simulink model "simulation_impulse"  (R2023b)
settings: Solver=VariableStepAuto  StartTime=0.0  StopTime=t_end  RelTol=1e-3
InitFcn:
  | param = plant_param();
undefined symbols (not defined in the file or in its folder): ue, xe
settings Model: Creator=block  LastModifiedBy=block

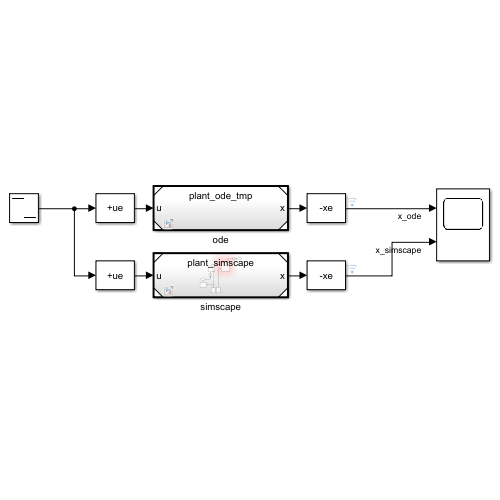
[thumbnail: Simulink's stored preview of the top-level diagram]
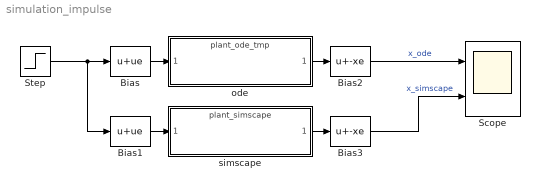
== system simulation_impulse ==
  Bias : Bias  Bias=ue  SaturateOnIntegerOverflow=off
  Bias1 : Bias  Bias=ue  SaturateOnIntegerOverflow=off
  Bias2 : Bias  Bias=-xe  SaturateOnIntegerOverflow=off
  Bias3 : Bias  Bias=-xe  SaturateOnIntegerOverflow=off
  Scope : Scope  NumInputPorts=2
  Step : Step  Time=0.01  Before=100  After=0  SampleTime=0
  ode : ModelReference  ModelNameDialog=plant_ode_tmp  SimulationMode=Normal  ModelReferenceVersion=1.2
  simscape : ModelReference  ModelNameDialog=plant_simscape  SimulationMode=Normal  ModelReferenceVersion=1.8
  wires:
  Bias2/1 -> Scope/1  "x_ode"
  Step/1 -> Bias/1, Bias1/1
  simscape/1 -> Bias3/1
  Bias/1 -> ode/1
  Bias1/1 -> simscape/1
  ode/1 -> Bias2/1
  Bias3/1 -> Scope/2  "x_simscape"
